simulink model "radial_compression"  (R2023b)
settings: Solver=ode45  StartTime=0.0  StopTime=Tstop  MaxStep=0.01  RelTol=1e-3
InitFcn:
  | init_params
values from neighbouring files (symbols this model uses):
  A0 = vessel.A0    [init_params.m]
  A_contact = 3e-4    (= 0.0003)    [init_params.m]
  alphaZ = 0.35    [init_params.m]
  Amin = vessel.Amin    [init_params.m]
  c1 = params.c1    [init_params.m]
  c2 = params.c2    [init_params.m]
  cc = params.cc    [init_params.m]
  eda_base = 0.15    [init_params.m]
  eda_gain = 0.8    [init_params.m]
  eda_noise_std = 0.0015    [init_params.m]
  eta = vessel.eta    [init_params.m]
  gamma = params.gamma    [init_params.m]
  heart_f = 1.2    [init_params.m]
  k1 = params.k1    [init_params.m]
  k2 = params.k2    [init_params.m]
  k_bleed = 0.08    [init_params.m]
  k_clot = 0.04    [init_params.m]
  kc = params.kc    [init_params.m]
  kPa2Pa = 1000    [init_params.m]
  m1 = params.m1    [init_params.m]
  m2 = params.m2    [init_params.m]
  P_art_amp = 2    [init_params.m]
  P_art_base = 16    [init_params.m]
  P_pain_scale = 16    [init_params.m]
  P_pain_th = 26    [init_params.m]
  Pc_noise_std = 0.015    [init_params.m]
  Pmax_kPa = 40    [init_params.m]    (also in make_protocolB.m = 25)
  ppg_drift_amp = 0.03    [init_params.m]
  ppg_drift_f = 0.05    [init_params.m]
  ppg_noise_std = 0.003    [init_params.m]
  Ps = vessel.Ps    [init_params.m]
  tau_dz = 1.5    [init_params.m]
  tau_eda = 3.5    [init_params.m]
  tau_env = 0.25    [init_params.m]
  tau_p = 0.5    [init_params.m]
  tau_pc_meas = 0.05    [init_params.m]
  tau_scl = 3.0    (= 3)    [init_params.m]
  trim_lim = 6    [init_params.m]
  Z0 = 1.0    (= 1)    [init_params.m]
  Z_noise_std = 0.002    [init_params.m]
undefined symbols (not defined in the file or in its folder): vessel
libraries: simulink x4, SignalEditorBlockLib x1
settings Model: Creator=17961  LastModifiedBy=17961

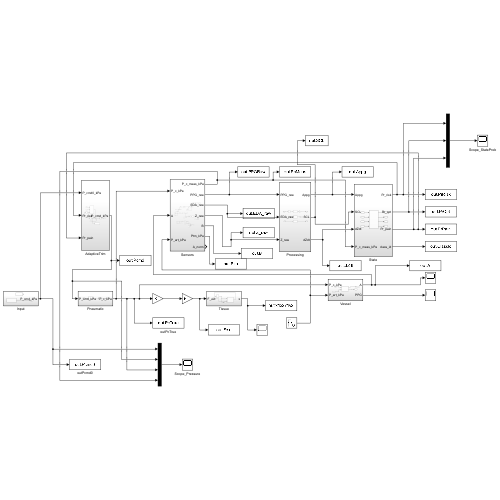
[thumbnail: Simulink's stored preview of the top-level diagram]
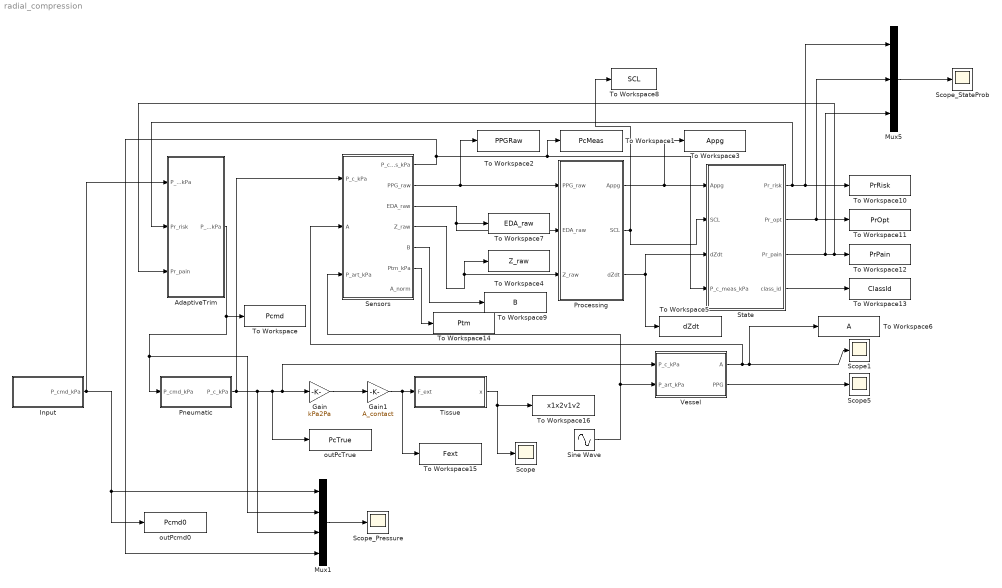
== system radial_compression ==
  AdaptiveTrim : Subsystem
  Gain : Gain  Gain=kPa2Pa
  Gain1 : Gain  Gain=A_contact
  Input : Subsystem
  Mux1 : Mux
  Mux5 : Mux  Inputs=3
  Pneumatic : Subsystem
  Processing : Subsystem
  Scope : Scope
  Scope1 : Scope
  Scope5 : Scope
  Scope_Pressure : Scope
  Scope_StateProb : Scope
  Sensors : Subsystem
  Sine Wave : Sin  Amplitude=P_art_amp  Bias=P_art_base  Frequency=2*pi*heart_f  SampleTime=0
  State : Subsystem
  Tissue : Subsystem
  To Workspace : ToWorkspace  VariableName=Pcmd  SaveFormat=Timeseries  SampleTime=-1
  To Workspace1 : ToWorkspace  VariableName=PcMeas  SaveFormat=Timeseries  SampleTime=-1
  To Workspace10 : ToWorkspace  VariableName=PrRisk  SaveFormat=Timeseries  SampleTime=-1
  To Workspace11 : ToWorkspace  VariableName=PrOpt  SaveFormat=Timeseries  SampleTime=-1
  To Workspace12 : ToWorkspace  VariableName=PrPain  SaveFormat=Timeseries  SampleTime=-1
  To Workspace13 : ToWorkspace  VariableName=ClassId  SaveFormat=Timeseries  SampleTime=-1
  To Workspace14 : ToWorkspace  VariableName=Ptm  SaveFormat=Timeseries  SampleTime=-1
  To Workspace15 : ToWorkspace  VariableName=Fext  SaveFormat=Timeseries  SampleTime=-1
  To Workspace16 : ToWorkspace  VariableName=x1x2v1v2  SaveFormat=Timeseries  SampleTime=-1
  To Workspace2 : ToWorkspace  VariableName=PPGRaw  SaveFormat=Timeseries  SampleTime=-1
  To Workspace3 : ToWorkspace  VariableName=Appg  SaveFormat=Timeseries  SampleTime=-1
  To Workspace4 : ToWorkspace  VariableName=Z_raw  SaveFormat=Timeseries  SampleTime=-1
  To Workspace5 : ToWorkspace  VariableName=dZdt  SaveFormat=Timeseries  SampleTime=-1
  To Workspace6 : ToWorkspace  VariableName=A  SaveFormat=Timeseries  SampleTime=-1
  To Workspace7 : ToWorkspace  VariableName=EDA_raw  SaveFormat=Timeseries  SampleTime=-1
  To Workspace8 : ToWorkspace  VariableName=SCL  SaveFormat=Timeseries  SampleTime=-1
  To Workspace9 : ToWorkspace  VariableName=B  SaveFormat=Timeseries  SampleTime=-1
  Vessel : Subsystem
  outPcTrue : ToWorkspace  VariableName=PcTrue  SaveFormat=Timeseries  SampleTime=-1
  outPcmd0 : ToWorkspace  VariableName=Pcmd0  SaveFormat=Timeseries  SampleTime=-1
  wires:
  Pneumatic/1(P_c_kPa) -> Sensors/1(P_c_kPa), Mux1/3, Gain/1, Vessel/1(P_c_kPa), outPcTrue/1
  Gain/1 -> Gain1/1
  Gain1/1 -> To Workspace15/1, Tissue/1(F_ext)
  Sine Wave/1 -> Sensors/3(P_art_kPa), Vessel/2(P_art_kPa)
  Input/1(P_cmd_kPa) -> outPcmd0/1, Mux1/1, AdaptiveTrim/1(P_cmd0_kPa)
  Tissue/1(x) -> To Workspace16/1, Scope/1
  Vessel/2(PPG) -> Scope5/1
  Vessel/1(A) -> Sensors/2(A), To Workspace6/1, Scope1/1
  Sensors/2(PPG_raw) -> Processing/1(PPG_raw), To Workspace2/1
  Sensors/3(EDA_raw) -> To Workspace7/1, Processing/2(EDA_raw)
  Sensors/4(Z_raw) -> Processing/3(Z_raw), To Workspace4/1
  Processing/1(Appg) -> To Workspace3/1, State/1(Appg)
  Processing/2(SCL) -> State/2(SCL), To Workspace8/1
  Processing/3(dZdt) -> To Workspace5/1, State/3(dZdt)
  Sensors/1(P_c_meas_kPa) -> Mux1/4, State/4(P_c_meas_kPa), To Workspace1/1
  State/1(Pr_risk) -> To Workspace10/1, Mux5/1, AdaptiveTrim/2(Pr_risk)
  State/3(Pr_pain) -> Mux5/3, AdaptiveTrim/3(Pr_pain), To Workspace12/1
  AdaptiveTrim/1(P_cmd_kPa) -> To Workspace/1, Mux1/2, Pneumatic/1(P_cmd_kPa)
  Sensors/5(B) -> To Workspace9/1
  State/2(Pr_opt) -> Mux5/2, To Workspace11/1
  State/4(class_id) -> To Workspace13/1
  Sensors/6(Ptm_kPa) -> To Workspace14/1
  Mux1/1 -> Scope_Pressure/1
  Mux5/1 -> Scope_StateProb/1

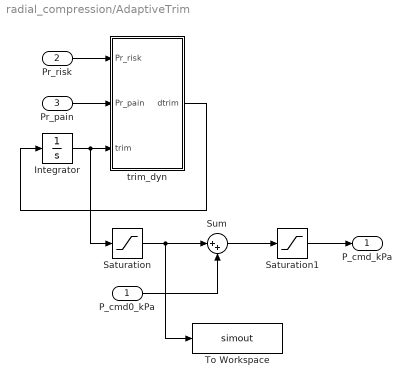
== system radial_compression/AdaptiveTrim ==
  P_cmd0_kPa : Inport
  Pr_risk : Inport  Port=2
  Pr_pain : Inport  Port=3
  Integrator : Integrator
  Saturation : Saturate  UpperLimit=trim_lim  LowerLimit=-trim_lim
  Saturation1 : Saturate  UpperLimit=Pmax_kPa  LowerLimit=0
  Sum : Sum  Inputs=|++
  To Workspace : ToWorkspace  VariableName=simout  SaveFormat=Timeseries  SampleTime=-1
  trim_dyn : MATLAB Function  TreatAsAtomicUnit=on
  P_cmd_kPa : Outport
  wires:
  Pr_risk/1 -> trim_dyn/1(Pr_risk)
  Pr_pain/1 -> trim_dyn/2(Pr_pain)
  Integrator/1 -> Saturation/1, trim_dyn/3(trim)
  trim_dyn/1(dtrim) -> Integrator/1
  Saturation/1 -> To Workspace/1, Sum/1
  P_cmd0_kPa/1 -> Sum/2
  Sum/1 -> Saturation1/1
  Saturation1/1 -> P_cmd_kPa/1

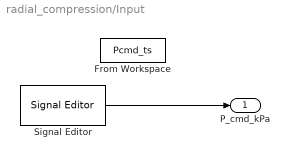
== system radial_compression/Input ==
  From Workspace : FromWorkspace  VariableName=Pcmd_ts  SampleTime=-1
  Signal Editor : SignalEditorBlockLib/Signal Editor  FileName=wave.mat  ActiveScenario=Scenario  ActiveSignal=P_cmd_kPa  IsBus=off  OutputBusObjectStr=Bus: BusObject  SampleTime=0  ZeroCross=off  OutputAfterFinalValue=Setting to zero  Unit=inherit  PreserveSignalName=on  ApplySigPropsToAllScenarios=on  ApplySigPropsToAllSignals=off
  P_cmd_kPa : Outport
  wires:
  Signal Editor/1 -> P_cmd_kPa/1

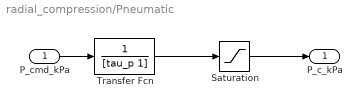
== system radial_compression/Pneumatic ==
  P_cmd_kPa : Inport
  Saturation : Saturate  UpperLimit=Pmax_kPa  LowerLimit=0
  Transfer Fcn : TransferFcn  Denominator=[tau_p 1]
  P_c_kPa : Outport
  wires:
  Transfer Fcn/1 -> Saturation/1
  P_cmd_kPa/1 -> Transfer Fcn/1
  Saturation/1 -> P_c_kPa/1

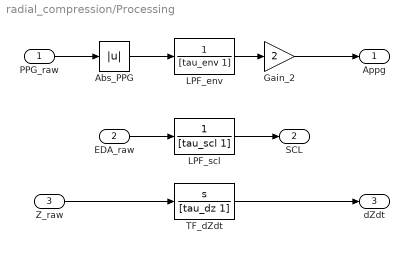
== system radial_compression/Processing ==
  PPG_raw : Inport
  EDA_raw : Inport  Port=2
  Z_raw : Inport  Port=3
  Abs_PPG : Abs  SaturateOnIntegerOverflow=off
  Gain_2 : Gain  Gain=2
  LPF_env : TransferFcn  Numerator=1  Denominator=[tau_env 1]
  LPF_scl : TransferFcn  Numerator=1  Denominator=[tau_scl 1]
  TF_dZdt : TransferFcn  Numerator=[1 0]  Denominator=[tau_dz 1]
  Appg : Outport
  SCL : Outport  Port=2
  dZdt : Outport  Port=3
  wires:
  PPG_raw/1 -> Abs_PPG/1
  Abs_PPG/1 -> LPF_env/1
  LPF_env/1 -> Gain_2/1
  Gain_2/1 -> Appg/1
  EDA_raw/1 -> LPF_scl/1
  LPF_scl/1 -> SCL/1
  Z_raw/1 -> TF_dZdt/1
  TF_dZdt/1 -> dZdt/1

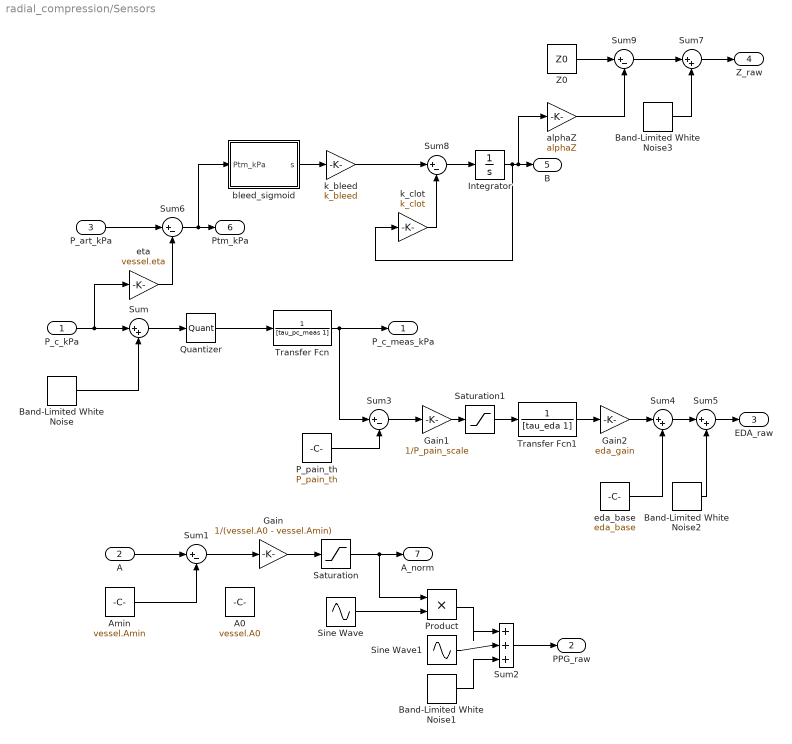
== system radial_compression/Sensors ==
  P_c_kPa : Inport
  A : Inport  Port=2
  P_art_kPa : Inport  Port=3
  A0 : Constant  Value=vessel.A0
  Amin : Constant  Value=vessel.Amin
  Band-Limited White Noise : simulink/Sources/Band-Limited White Noise  Cov=Pc_noise_std^2  Ts=0.001  seed=[23341]
  Band-Limited White Noise1 : simulink/Sources/Band-Limited White Noise  Cov=ppg_noise_std^2  Ts=0.001  seed=[23341]
  Band-Limited White Noise2 : simulink/Sources/Band-Limited White Noise  Cov=eda_noise_std^2  Ts=0.001  seed=[23341]
  Band-Limited White Noise3 : simulink/Sources/Band-Limited White Noise  Cov=Z_noise_std^2  Ts=0.001  seed=[23341]
  Gain : Gain  Gain=1/(vessel.A0 - vessel.Amin)
  Gain1 : Gain  Gain=1/P_pain_scale
  Gain2 : Gain  Gain=eda_gain
  Integrator : Integrator  InitialCondition=0.05
  P_pain_th : Constant  Value=P_pain_th
  Product : Product
  Quantizer : Quantizer  QuantizationInterval=Pc_quant_step
  Saturation : Saturate  UpperLimit=1  LowerLimit=0
  Saturation1 : Saturate  UpperLimit=1  LowerLimit=0
  Sine Wave : Sin  Frequency=2*pi*heart_f  SampleTime=0
  Sine Wave1 : Sin  Amplitude=ppg_drift_amp  Frequency=2*pi*ppg_drift_f  SampleTime=0
  Sum{,4..5,7} (4 alike) : Sum  Inputs=|++
  Sum{1,3,6,8..9} (5 alike) : Sum  Inputs=|+-
  Sum2 : Sum  Inputs=|+++
  Transfer Fcn : TransferFcn  Numerator=1  Denominator=[tau_pc_meas 1]
  Transfer Fcn1 : TransferFcn  Numerator=1  Denominator=[tau_eda 1]
  Z0 : Constant  Value=Z0
  alphaZ : Gain  Gain=alphaZ
  bleed_sigmoid : MATLAB Function  TreatAsAtomicUnit=on
  eda_base : Constant  Value=eda_base
  eta : Gain  Gain=vessel.eta
  k_bleed : Gain  Gain=k_bleed
  k_clot : Gain  Gain=k_clot
  P_c_meas_kPa : Outport
  PPG_raw : Outport  Port=2
  EDA_raw : Outport  Port=3
  Z_raw : Outport  Port=4
  B : Outport  Port=5
  Ptm_kPa : Outport  Port=6
  A_norm : Outport  Port=7
  wires:
  P_c_kPa/1 -> Sum/1, eta/1
  Band-Limited White Noise/1 -> Sum/2
  Quantizer/1 -> Transfer Fcn/1
  Transfer Fcn/1 -> Sum3/1, P_c_meas_kPa/1
  Sum/1 -> Quantizer/1
  A/1 -> Sum1/1
  Amin/1 -> Sum1/2
  Sum1/1 -> Gain/1
  Gain/1 -> Saturation/1
  Saturation/1 -> Product/1, A_norm/1
  Sine Wave/1 -> Product/2
  Product/1 -> Sum2/1
  Sine Wave1/1 -> Sum2/2
  Band-Limited White Noise1/1 -> Sum2/3
  Sum2/1 -> PPG_raw/1
  Sum3/1 -> Gain1/1
  Gain1/1 -> Saturation1/1
  Saturation1/1 -> Transfer Fcn1/1
  Transfer Fcn1/1 -> Gain2/1
  Gain2/1 -> Sum4/1
  Sum4/1 -> Sum5/1
  Band-Limited White Noise2/1 -> Sum5/2
  Sum5/1 -> EDA_raw/1
  P_pain_th/1 -> Sum3/2
  eda_base/1 -> Sum4/2
  P_art_kPa/1 -> Sum6/1
  eta/1 -> Sum6/2
  Sum6/1 -> bleed_sigmoid/1(Ptm_kPa), Ptm_kPa/1
  bleed_sigmoid/1(s) -> k_bleed/1
  Integrator/1 -> k_clot/1, alphaZ/1, B/1
  k_bleed/1 -> Sum8/1
  k_clot/1 -> Sum8/2
  Sum8/1 -> Integrator/1
  Z0/1 -> Sum9/1
  alphaZ/1 -> Sum9/2
  Sum9/1 -> Sum7/1
  Band-Limited White Noise3/1 -> Sum7/2
  Sum7/1 -> Z_raw/1

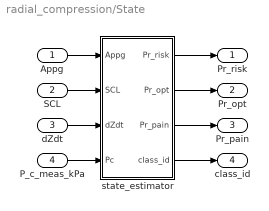
== system radial_compression/State ==
  Appg : Inport
  SCL : Inport  Port=2
  dZdt : Inport  Port=3
  P_c_meas_kPa : Inport  Port=4
  state_estimator : MATLAB Function  TreatAsAtomicUnit=on
  Pr_risk : Outport
  Pr_opt : Outport  Port=2
  Pr_pain : Outport  Port=3
  class_id : Outport  Port=4
  wires:
  Appg/1 -> state_estimator/1(Appg)
  SCL/1 -> state_estimator/2(SCL)
  dZdt/1 -> state_estimator/3(dZdt)
  P_c_meas_kPa/1 -> state_estimator/4(Pc)
  state_estimator/1(Pr_risk) -> Pr_risk/1
  state_estimator/2(Pr_opt) -> Pr_opt/1
  state_estimator/3(Pr_pain) -> Pr_pain/1
  state_estimator/4(class_id) -> class_id/1

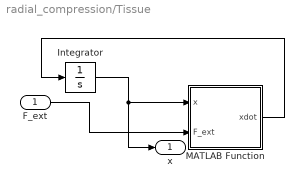
== system radial_compression/Tissue ==
  F_ext : Inport
  Integrator : Integrator  InitialCondition=[0;0;0;0]
  MATLAB Function : MATLAB Function  TreatAsAtomicUnit=on
  x : Outport
  wires:
  Integrator/1 -> x/1, MATLAB Function/1(x)
  F_ext/1 -> MATLAB Function/2(F_ext)
  MATLAB Function/1(xdot) -> Integrator/1

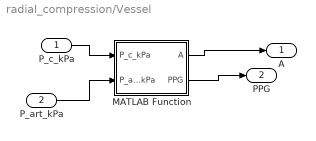
== system radial_compression/Vessel ==
  P_c_kPa : Inport
  P_art_kPa : Inport  Port=2
  MATLAB Function : MATLAB Function  TreatAsAtomicUnit=on
  A : Outport
  PPG : Outport  Port=2
  wires:
  MATLAB Function/1(A) -> A/1
  MATLAB Function/2(PPG) -> PPG/1
  P_c_kPa/1 -> MATLAB Function/1(P_c_kPa)
  P_art_kPa/1 -> MATLAB Function/2(P_art_kPa)

== matlab function radial_compression/Vessel/MATLAB Function ==
  data: P_c_kPa input; A output; P_art_kPa input; PPG output; eta parameter double size=[1 1]; A0 parameter double size=[1 1]; Amin parameter double size=[1 1]; Ps parameter double size=[1 1]
function [A, PPG] = vessel_map(P_c_kPa, P_art_kPa, eta, A0, Amin, Ps)
% 用标量参数：eta, A0, Amin, Ps（在工作区定义，并在 Symbols 里设为 Parameter）

% 等效外压（kPa）
Pext = eta * P_c_kPa;

% 跨壁压（kPa）
Ptm = P_art_kPa - Pext;

% sigmoid 映射到归一化截面积 A
A = Amin + (A0 - Amin) / (1 + exp(-Ptm / Ps));

% PPG（示意）：截面积去一个常量偏置
PPG = A - 0.5*(A0 + Amin);

== matlab function radial_compression/Tissue/MATLAB Function ==
  data: x input double size=[4 1]; xdot output double size=[4 1]; F_ext input; m1 parameter double size=[1 1]; m2 parameter double size=[1 1]; k1 parameter double size=[1 1]; k2 parameter double size=[1 1]; c1 parameter double size=[1 1]; c2 parameter double size=[1 1]; kc parameter double size=[1 1]; cc parameter double size=[1 1]; gamma parameter double size=[1 1]
function xdot = tissue_ode(x, F_ext, m1, m2, k1, k2, c1, c2, kc, cc, gamma)
% x = [x1; v1; x2; v2]
% F_ext: 外力(N)

% ---- 状态 ----
x1 = x(1); v1 = x(2);
x2 = x(3); v2 = x(4);

% ---- 这里直接用工作区变量：m1,m2,k1,k2,c1,c2,kc,cc,gamma ----
% 关键：这些变量下一步要在 Symbols 里设置为 Parameter

% 耦合力
F_couple = kc*(x1 - x2) + cc*(v1 - v2);

% 表层（可选轻非线性硬化）
F_k1 = k1*x1 + gamma*x1^3;
F_c1 = c1*v1;

% 深层（线性）
F_k2 = k2*x2;
F_c2 = c2*v2;

% 加速度
a1 = (F_ext - F_k1 - F_c1 - F_couple) / m1;
a2 = (F_couple - F_k2 - F_c2) / m2;

% 输出导数（4×1）
xdot = [v1; a1; v2; a2];

== matlab function radial_compression/Sensors/bleed_sigmoid ==
  data: Ptm_kPa input; s output
function s = bleed_sigmoid(Ptm_kPa)

P_bleed_th    = 8;
P_bleed_slope = 2;

u = (Ptm_kPa - P_bleed_th) / P_bleed_slope;
s = 1 / (1 + exp(-u));

== matlab function radial_compression/State/state_estimator ==
  data: Appg input; Pr_risk output; SCL input; dZdt input; Pc input; Pr_opt output; Pr_pain output; class_id output
function [Pr_risk, Pr_opt, Pr_pain, class_id] = state_estimator(Appg, SCL, dZdt, Pc)

% ===== 先把参数直接写死，先跑通 =====
Appg_low    = 0.15;
P_pain_th   = 18;
P_pain_scale= 10;

wZ   = 3;
wPPG = 2;
wSCL = 2;
wP   = 1;
w0   = 1;

% ===== 特征构造 =====
% 出血：阻抗下降 => dZdt < 0，因此用 -dZdt
risk_feat = max(0, -dZdt);

% 灌注低：Appg低于阈值越多越危险
ppg_feat = max(0, Appg_low - Appg);

% 疼痛：压力高于阈值
pain_feat = max(0, (Pc - P_pain_th)/P_pain_scale);

% ===== 三类分数 =====
s_risk = wZ*risk_feat + wPPG*ppg_feat;
s_pain = wSCL*SCL + wP*pain_feat;
s_opt  = w0;

% ===== softmax 概率 =====
m = max([s_risk, s_opt, s_pain]);
e = exp([s_risk, s_opt, s_pain] - m);
p = e / sum(e);

Pr_risk = p(1);
Pr_opt  = p(2);
Pr_pain = p(3);

% 1=risk, 2=opt, 3=pain
[~, class_id] = max([Pr_risk, Pr_opt, Pr_pain]);

== matlab function radial_compression/AdaptiveTrim/trim_dyn ==
  data: Pr_risk input; dtrim output; Pr_pain input; trim input
function dtrim = trim_dyn(Pr_risk, Pr_pain, trim)

trim_enable = 1;
k_trim_up   = 0.8;
k_trim_dn   = 0.8;
tau_trim    = 1.0;

u = k_trim_up*(Pr_risk - 0.33) - k_trim_dn*(Pr_pain - 0.33);
dtrim = (u - trim) / tau_trim;

if trim_enable == 0
    dtrim = -trim / tau_trim;
end
